simulink model "InverseController"  (R2022b)
settings: Solver=VariableStepAuto  StartTime=0.0  StopTime=30.0  RelTol=1e-3
values from neighbouring files (symbols this model uses):
  f = 0.5    [parameters.m]
settings Model: Creator=eleves  LastModifiedBy=eleves
settings ModelReferenceCC: EnableRefExpFcnMdlSchedulingChecks=on

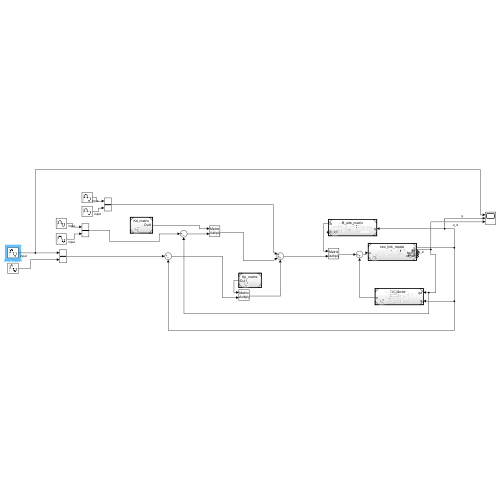
[thumbnail: Simulink's stored preview of the top-level diagram]
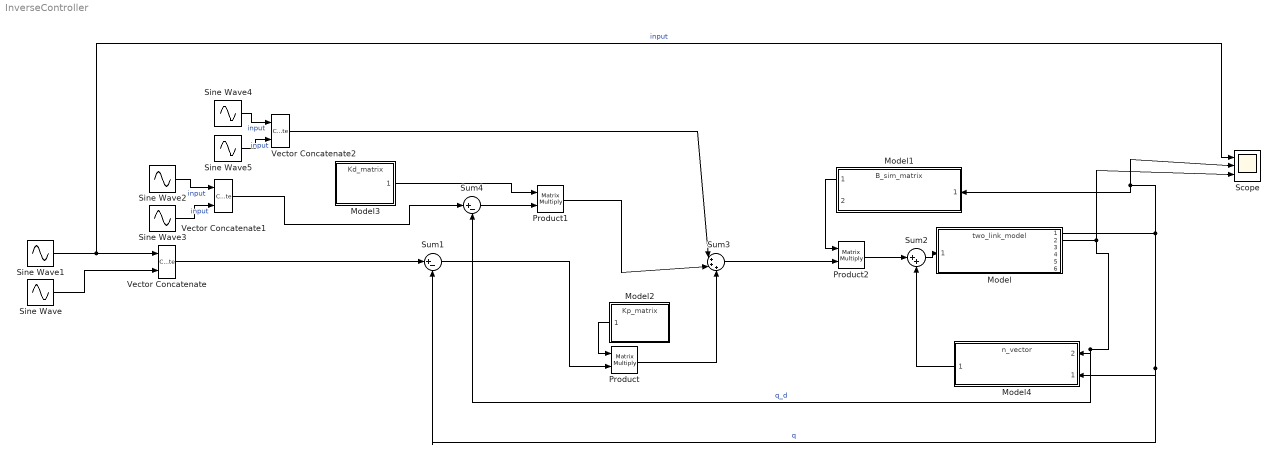
== system InverseController ==
  Model : ModelReference  ModelNameDialog=two_link_model.slx  SimulationMode=Normal  ModelReferenceVersion=13.58
  Model1 : ModelReference  ModelNameDialog=B_sim_matrix.slx  SimulationMode=Normal  ModelReferenceVersion=1.6
  Model2 : ModelReference  ModelNameDialog=Kp_matrix.slx  SimulationMode=Normal  ModelReferenceVersion=1.3
  Model3 : ModelReference  ModelNameDialog=Kd_matrix.slx  SimulationMode=Normal  ModelReferenceVersion=1.2
  Model4 : ModelReference  ModelNameDialog=n_vector.slx  SimulationMode=Normal  ModelReferenceVersion=1.3
      settings: PortSchema="{\"entries\":[{\"content\":{\"sides\":[{\"content\":{\"connectorIds\":[\"In2\",\"In1\"]},\"type\":\"ConnectorPlacement.EquallySpacedRectSide\",\"uuid\":\"0004a852-6b57-412e-a247-f7a948c02aef\"},{\"content\":{\"connectorIds\":[\"Out1\"],\"side\":\"RIGHT\"},\"type\":\"ConnectorPlacement.EquallySpacedRectSide\",\"uuid\":\"2c6a1f56-b264-4a50-8175-f4e8d5862eda\"},{\"content\":{\"connectorIds\":[],\"side\":\"TOP\"},\"type\":\"ConnectorPlacement.EquallySpacedRectSide\",\"uuid\":\"b3451316-5974-4a81-98c7-74555a3ec881\"}]},\"type\":\"ConnectorPlacement.EquallySpacedConnector\",\"uuid\":\"ac2390f0-df41-4187-a0e3-0c9a5394d303\"}],\"packageUris\":[\"http://schema.mathworks.com/mf0/Connector/R2020b\"],\"version\":\"1.0\"}"
  Product : Product  Multiplication=Matrix(*)
  Product1 : Product  Multiplication=Matrix(*)
  Product2 : Product  Multiplication=Matrix(*)
  Scope : Scope  NumInputPorts=3
  Sine Wave : Sin  Frequency=f  SampleTime=0.01
  Sine Wave1 : Sin  Frequency=f  SampleTime=0.01
  Sine Wave2 : Sin  Amplitude=2*pi*f  Frequency=f  Phase=pi/2  SampleTime=0.01
  Sine Wave3 : Sin  Amplitude=2*pi*f  Frequency=f  Phase=pi/2  SampleTime=0.01
  Sine Wave4 : Sin  Amplitude=-(2*pi*f)^2  Frequency=f  SampleTime=0.01
  Sine Wave5 : Sin  Amplitude=-(2*pi*f)^2  Frequency=f  SampleTime=0.01
  Sum1 : Sum  Inputs=|+-
  Sum2 : Sum  Inputs=|++
  Sum3 : Sum  Inputs=|+++
  Sum4 : Sum  Inputs=|+-
  Vector Concatenate : Concatenate
  Vector Concatenate1 : Concatenate
  Vector Concatenate2 : Concatenate
  wires:
  Sine Wave1/1 -> Scope/1, Vector Concatenate/1  "input"
  Sine Wave/1 -> Vector Concatenate/2
  Sum2/1 -> Model/1
  Model/1 -> Scope/2, Model1/1, Sum1/2, Model4/1  "q"
  Model2/1 -> Product/1
  Sum1/1 -> Product/2
  Vector Concatenate/1 -> Sum1/1
  Model3/1 -> Product1/1
  Model/2 -> Sum4/2, Model4/2, Scope/3  "q_d"
  Product2/1 -> Sum2/1
  Product/1 -> Sum3/3
  Sum4/1 -> Product1/2
  Product1/1 -> Sum3/2
  Model4/1 -> Sum2/2
  Model1/1 -> Product2/1
  Sum3/1 -> Product2/2
  Sine Wave2/1 -> Vector Concatenate1/1  "input"
  Sine Wave3/1 -> Vector Concatenate1/2  "input"
  Vector Concatenate1/1 -> Sum4/1
  Sine Wave4/1 -> Vector Concatenate2/1  "input"
  Sine Wave5/1 -> Vector Concatenate2/2  "input"
  Vector Concatenate2/1 -> Sum3/1
